simulink model "simulation_of_single_ph_transformer"  (R2014b)
settings: Solver=ode23tb  StartTime=0.0  StopTime=0.2  MaxStep=1e-4  RelTol=1e-3
libraries: powerlib x8, powerlib_meascontrol x4
settings Model: Creator=Amr Saleh  LastModifiedBy=Amr Saleh

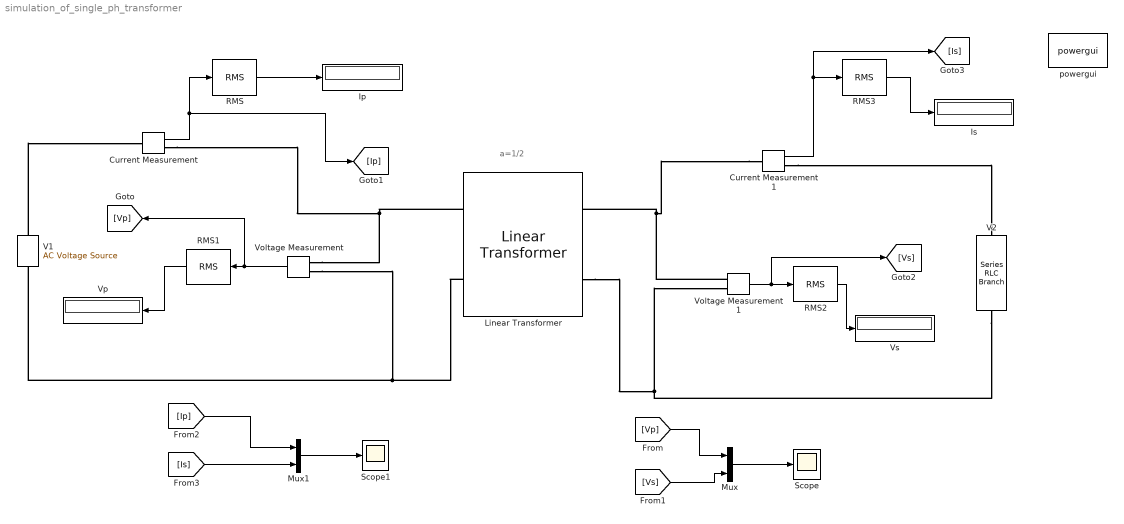
== system simulation_of_single_ph_transformer ==
  note: a=1/2
  Current Measurement : powerlib/Measurements/Current Measurement  PhasorSimulation=off  OutputType=Complex  PSBequivalent=0
  Current Measurement1 : powerlib/Measurements/Current Measurement  PhasorSimulation=off  OutputType=Complex  PSBequivalent=0
  Ip : Display
  Is : Display
  Linear Transformer : powerlib/Elements/Linear Transformer  UNITS=pu  NominalPower=[ 2e6 50 ]  winding1="[ 400  0.002  0.08 ]"  winding2="[ 800  0.002  0.08 ]"  ThreeWindings=off  winding3=[ 315e3 0.002 0.08 ]  RmLm=[ 4000 4000 ]  Measurements=None  DataType=off
  Mux : Mux  Inputs=2
  Mux1 : Mux  Inputs=2
  RMS{,1..3} (4 alike) : powerlib_meascontrol/Measurements/RMS  TrueRMS=off  Freq=50  RMSInit=0  Ts=0
  Scope : Scope
  Scope1 : Scope
  V1 : powerlib/Electrical Sources/AC Voltage Source  Amplitude=220*sqrt(2)  Phase=0  Frequency=50  SampleTime=0  Measurements=None
  V2 : powerlib/Elements/Series RLC Branch  LConnTagsString=__new0  RConnTagsString=__new0  BranchType=R  Resistance=10  Inductance=1e-3  SetiL0=off  InitialCurrent=0  Capacitance=1e-6  Setx0=off  InitialVoltage=0  Measurements=None
  Voltage Measurement : powerlib/Measurements/Voltage Measurement  PhasorSimulation=off  OutputType=Complex  PSBequivalent=0
  Voltage Measurement1 : powerlib/Measurements/Voltage Measurement  PhasorSimulation=off  OutputType=Complex  PSBequivalent=0
  Vp : Display
  Vs : Display
  powergui : powerlib/powergui  Priority=1  SimulationMode=Continuous  SolverType=Tustin/Backward Euler (TBE)  SampleTime=50e-6  frequency=60  SPID=off  DisableSnubberDevices=off  DisableRonSwitches=off  DisableVfSwitches=off  SwTol=0  DisplayEquations=off  Interpol=off  methode=off  Ts=100  frequencyindice=50  Pbase=100e6  ErrMax=1e-4  Iterations=50  UnitsV=kV  UnitsW=MW  FunctionMessages=off  echomessages=off  HookPort=off  EnableUseOfTLC=off  x0status=blocks  RestoreLinks=warning  ResistiveCurrentMeasurement=off  Frange=[0:2:500]  Ylog=off  Xlog=on  ShowGrid=off  save=off  variable=ZData  structure=0  ZoomFFT=off  StartTime=0.0  cycles=1  DisplayStyle=1  fundamental=60  FreqAxis=off  MaxFrequency=1000  frequencyindicesteady=1  RmsSteady=1  display=off
  wires:
  Current Measurement/1 -> [Ip], RMS/1
  RMS/1 -> Ip/1
  Voltage Measurement/1 -> [Vp], RMS1/1
  RMS1/1 -> Vp/1
  Voltage Measurement1/1 -> [Vs], RMS2/1
  RMS2/1 -> Vs/1
  Current Measurement1/1 -> [Is], RMS3/1
  RMS3/1 -> Is/1
  Mux/1 -> Scope/1
  [Vp] -> Mux/1
  [Vs] -> Mux/2
  Mux1/1 -> Scope1/1
  [Ip] -> Mux1/1
  [Is] -> Mux1/2
  connections:
  V1/RConn1 -- Current Measurement/LConn1
  Current Measurement/RConn1 -- Voltage Measurement/LConn1 -- Linear Transformer/LConn1
  Voltage Measurement/LConn2 -- Linear Transformer/LConn2 -- V1/LConn1
  Current Measurement1/LConn1 -- Linear Transformer/RConn1 -- Voltage Measurement1/LConn1
  Current Measurement1/RConn1 -- V2/LConn1
  V2/RConn1 -- Linear Transformer/RConn2 -- Voltage Measurement1/LConn2
